simulink model "dft_polyphase_channelizer_4_by_2"  (R2018b)
settings: Solver=FixedStepDiscrete  StartTime=0.0  StopTime=t(end)  RelTol=1e-3  EnableMultiTasking=on
InitFcn:
  | M = 4; % Number of channels in the filter bank.
  | N = 8;  % Number of taps in each FIR filter.
  | n_out = 4000; % Number of output samples
  | datatypeselector = 'dsp'; % 'double' 'single' 'hdl' 'dsp'
  | fidatatype = 'Fixed'; % 'Fixed' 'ScaledDouble'
  | [T,B,U,b,u,t,fs] = generate_inputs(M,N,n_out,datatypeselector,fidatatype);
undefined symbols (not defined in the file or in its folder): B, fs, T
settings Model: Creator=tbryan  LastModifiedBy=tbryan
settings SolverCC: AutoInsertRateTranBlk=on
settings OptimizationCC: LifeSpan=inf
settings DebuggingCC: AllowSymbolicDim=off  LibraryContextMissingDiagnostic=none  SFUnexpectedBacktrackingDiag=warning  SFNoUnconditionalDefaultTransitionDiag=warning  SFExecutionAtInitializationDiag=none
settings SFSimCC: SimUseLocalCustomCode=off
settings RTWCC: RTWUseLocalCustomCode=off
settings CodeAppCC: StateflowObjectComments=on
settings GRTTargetCC: TargetLangStandard=C89/C90 (ANSI)  GeneratePreprocessorConditionals=Disable all
settings ConfigComp: CovMetricSettings=dw  CovHtmlReporting=on  CovSaveCumulativeToWorkspaceVar=on  CovSaveSingleToWorkspaceVar=on  CovExternalEMLEnable=off

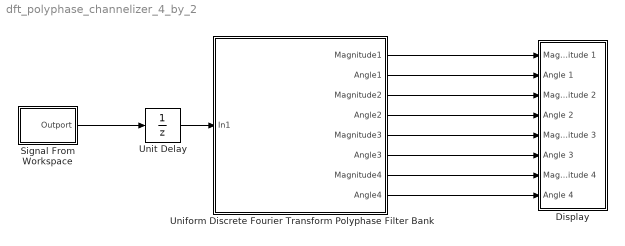
== system dft_polyphase_channelizer_4_by_2 ==
  Display : Subsystem
  Signal From Workspace : Subsystem  mask(Signal From Workspace){X=u, Ts=1/fs, nsamps=1, OutputAfterFinalValue=Setting to zero, ignoreOrWarnInputAndFrameLengths=off, OutputFrames=off}
      mask prompts: X "Signal:"; Ts "Sample time:"; nsamps "Samples per frame:"; OutputAfterFinalValue "Form output after final data value by:"; ignoreOrWarnInputAndFrameLengths "Warn when frame size does not evenly divide input length"; OutputFrames "Output Frames"
      mask help:
      | Output signal samples obtained from the MATLAB workspace at successive sample times.  A signal matrix is interpreted as having one channel per column.  Signal columns may be buffered into frames by specifying a number of samples per frame greater than 1.
      |
      | An M x N x P signal array outputs M x N matrices at successive sample times.  The samples per frame must be equal to 1 for three-dimensional signal arrays.
      mask init:
      | dispX = get_param(gcbh, 'X');
      | [s,Ts] = dspblksfw2('init', X,Ts,nsamps);
      mask Help: eval('blocksethelp');
      mask TypeOptions OutputAfterFinalValue: Setting to zero | Holding final value | Cyclic repetition
      mask Callback OutputAfterFinalValue: dspblksfw2
      mask Display: disp(dispX)
  Uniform Discrete Fourier Transform Polyphase Filter Bank : Subsystem
  Unit Delay : UnitDelay  SampleTime=-1
  wires:
  Signal From Workspace/1(Outport) -> Unit Delay/1
  Unit Delay/1 -> Uniform Discrete Fourier Transform Polyphase Filter Bank/1(In1)
  Uniform Discrete Fourier Transform Polyphase Filter Bank/1(Magnitude1) -> Display/1(Magnitude 1)
  Uniform Discrete Fourier Transform Polyphase Filter Bank/2(Angle1) -> Display/2(Angle 1)
  Uniform Discrete Fourier Transform Polyphase Filter Bank/3(Magnitude2) -> Display/3(Magnitude 2)
  Uniform Discrete Fourier Transform Polyphase Filter Bank/4(Angle2) -> Display/4(Angle 2)
  Uniform Discrete Fourier Transform Polyphase Filter Bank/5(Magnitude3) -> Display/5(Magnitude 3)
  Uniform Discrete Fourier Transform Polyphase Filter Bank/6(Angle3) -> Display/6(Angle 3)
  Uniform Discrete Fourier Transform Polyphase Filter Bank/7(Magnitude4) -> Display/7(Magnitude 4)
  Uniform Discrete Fourier Transform Polyphase Filter Bank/8(Angle4) -> Display/8(Angle 4)

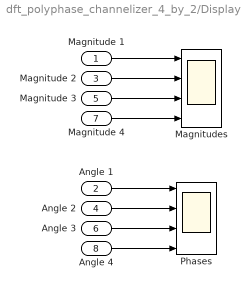
== system dft_polyphase_channelizer_4_by_2/Display ==
  Magnitude 1 : Inport
  Angle 1 : Inport  Port=2
  Magnitude 2 : Inport  Port=3
  Angle 2 : Inport  Port=4
  Magnitude 3 : Inport  Port=5
  Angle 3 : Inport  Port=6
  Magnitude 4 : Inport  Port=7
  Angle 4 : Inport  Port=8
  Magnitudes : Scope  NumInputPorts=4
  Phases : Scope  NumInputPorts=4
  wires:
  Angle 3/1 -> Phases/3
  Magnitude 2/1 -> Magnitudes/2
  Magnitude 1/1 -> Magnitudes/1
  Magnitude 4/1 -> Magnitudes/4
  Angle 2/1 -> Phases/2
  Angle 4/1 -> Phases/4
  Magnitude 3/1 -> Magnitudes/3
  Angle 1/1 -> Phases/1

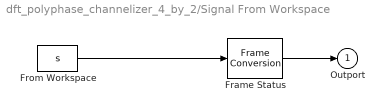
== system dft_polyphase_channelizer_4_by_2/Signal From Workspace ==
  Frame Status : FrameConversion  OutFrame=Sample-based
  From Workspace : FromWorkspace  VariableName=s  SampleTime=Ts  Interpolate=off  OutputAfterFinalValue=Setting to zero
  Outport : Outport  InitialOutput=0
  wires:
  Frame Status/1 -> Outport/1
  From Workspace/1 -> Frame Status/1

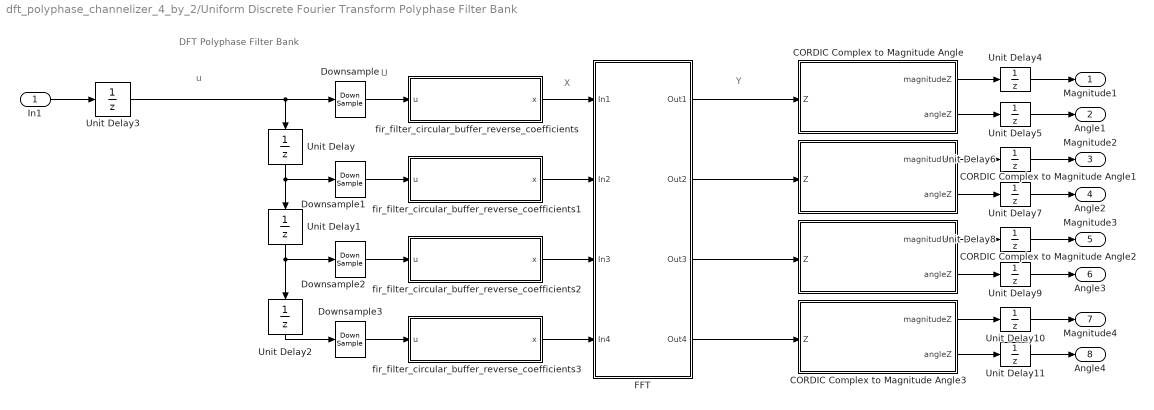
== system dft_polyphase_channelizer_4_by_2/Uniform Discrete Fourier Transform Polyphase Filter Bank ==
  note: DFT Polyphase Filter Bank
  note: U
  note: u
  note: X
  note: Y
  In1 : Inport
  " CORDIC Complex to Magnitude Angle" : MATLAB Function  TreatAsAtomicUnit=on
  " CORDIC Complex to Magnitude Angle1" : MATLAB Function  TreatAsAtomicUnit=on
  " CORDIC Complex to Magnitude Angle2" : MATLAB Function  TreatAsAtomicUnit=on
  " CORDIC Complex to Magnitude Angle3" : MATLAB Function  TreatAsAtomicUnit=on
  Downsample{,1..3} (4 alike) : DownSample  N=4  RateOptions=Allow multirate processing
  FFT : Subsystem
      mask Display: disp('IDFT')
  Unit Delay{,1..11} (12 alike) : UnitDelay  SampleTime=-1
  fir_filter_circular_buffer_reverse_coefficients : MATLAB Function  TreatAsAtomicUnit=on  mask{b=B(1,:), T=T.fir_filter}
      mask prompts: b "Coefficients: b from MATLAB's filter(b,1,x)"
  fir_filter_circular_buffer_reverse_coefficients1 : MATLAB Function  TreatAsAtomicUnit=on  mask{b=B(2,:), T=T.fir_filter}
      mask prompts: b "Coefficients: b from MATLAB's filter(b,1,x)"
  fir_filter_circular_buffer_reverse_coefficients2 : MATLAB Function  TreatAsAtomicUnit=on  mask{b=B(3,:), T=T.fir_filter}
      mask prompts: b "Coefficients: b from MATLAB's filter(b,1,x)"
  fir_filter_circular_buffer_reverse_coefficients3 : MATLAB Function  TreatAsAtomicUnit=on  mask{b=B(4,:), T=T.fir_filter}
      mask prompts: b "Coefficients: b from MATLAB's filter(b,1,x)"
  Magnitude1 : Outport
  Angle1 : Outport  Port=2
  Magnitude2 : Outport  Port=3
  Angle2 : Outport  Port=4
  Magnitude3 : Outport  Port=5
  Angle3 : Outport  Port=6
  Magnitude4 : Outport  Port=7
  Angle4 : Outport  Port=8
  wires:
  FFT/1(Out1) -> " CORDIC Complex to Magnitude Angle"/1(Z)
  FFT/2(Out2) -> " CORDIC Complex to Magnitude Angle1"/1(Z)
  FFT/3(Out3) -> " CORDIC Complex to Magnitude Angle2"/1(Z)
  FFT/4(Out4) -> " CORDIC Complex to Magnitude Angle3"/1(Z)
  Unit Delay1/1 -> Unit Delay2/1, Downsample2/1
  fir_filter_circular_buffer_reverse_coefficients1/1(x) -> FFT/2(In2)
  Unit Delay/1 -> Unit Delay1/1, Downsample1/1
  fir_filter_circular_buffer_reverse_coefficients/1(x) -> FFT/1(In1)
  fir_filter_circular_buffer_reverse_coefficients2/1(x) -> FFT/3(In3)
  Unit Delay2/1 -> Downsample3/1
  fir_filter_circular_buffer_reverse_coefficients3/1(x) -> FFT/4(In4)
  Downsample3/1 -> fir_filter_circular_buffer_reverse_coefficients3/1(u)
  Downsample2/1 -> fir_filter_circular_buffer_reverse_coefficients2/1(u)
  Downsample1/1 -> fir_filter_circular_buffer_reverse_coefficients1/1(u)
  Downsample/1 -> fir_filter_circular_buffer_reverse_coefficients/1(u)
  In1/1 -> Unit Delay3/1
  Unit Delay3/1 -> Unit Delay/1, Downsample/1
  Unit Delay4/1 -> Magnitude1/1
  " CORDIC Complex to Magnitude Angle"/1(magnitudeZ) -> Unit Delay4/1
  Unit Delay5/1 -> Angle1/1
  " CORDIC Complex to Magnitude Angle"/2(angleZ) -> Unit Delay5/1
  Unit Delay6/1 -> Magnitude2/1
  " CORDIC Complex to Magnitude Angle1"/1(magnitudeZ) -> Unit Delay6/1
  Unit Delay7/1 -> Angle2/1
  " CORDIC Complex to Magnitude Angle1"/2(angleZ) -> Unit Delay7/1
  Unit Delay8/1 -> Magnitude3/1
  " CORDIC Complex to Magnitude Angle2"/1(magnitudeZ) -> Unit Delay8/1
  Unit Delay9/1 -> Angle3/1
  " CORDIC Complex to Magnitude Angle2"/2(angleZ) -> Unit Delay9/1
  Unit Delay10/1 -> Magnitude4/1
  " CORDIC Complex to Magnitude Angle3"/1(magnitudeZ) -> Unit Delay10/1
  Unit Delay11/1 -> Angle4/1
  " CORDIC Complex to Magnitude Angle3"/2(angleZ) -> Unit Delay11/1

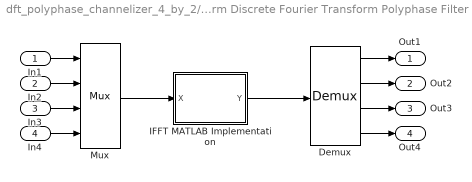
== system dft_polyphase_channelizer_4_by_2/Uniform Discrete Fourier Transform Polyphase Filter Bank/FFT ==
  In1 : Inport
  In2 : Inport  Port=2
  In3 : Inport  Port=3
  In4 : Inport  Port=4
  Demux : Demux
  IFFT MATLAB Implementation : MATLAB Function  TreatAsAtomicUnit=on  mask{T=T.fft}
      mask prompts: T "Types table"
  Mux : Mux
  Out1 : Outport
  Out2 : Outport  Port=2
  Out3 : Outport  Port=3
  Out4 : Outport  Port=4
  wires:
  Mux/1 -> IFFT MATLAB Implementation/1(X)
  IFFT MATLAB Implementation/1(Y) -> Demux/1
  In1/1 -> Mux/1
  In4/1 -> Mux/4
  In3/1 -> Mux/3
  In2/1 -> Mux/2
  Demux/2 -> Out2/1
  Demux/3 -> Out3/1
  Demux/4 -> Out4/1
  Demux/1 -> Out1/1

== matlab function dft_polyphase_channelizer_4_by_2/Uniform Discrete Fourier Transform Polyphase Filter Bank/ CORDIC Complex to Magnitude Angle1 ==
  data: Z input; magnitudeZ output; angleZ output
function [magnitudeZ, angleZ] = cordic_magnitude_angle(Z)
    [magnitudeZ, angleZ] = cordic_cart2pol(Z);
end

== matlab function dft_polyphase_channelizer_4_by_2/Uniform Discrete Fourier Transform Polyphase Filter Bank/ CORDIC Complex to Magnitude Angle ==
  data: Z input; magnitudeZ output; angleZ output
function [magnitudeZ, angleZ] = cordic_magnitude_angle(Z)
    [magnitudeZ, angleZ] = cordic_cart2pol(Z);
end

== matlab function dft_polyphase_channelizer_4_by_2/Uniform Discrete Fourier Transform Polyphase Filter Bank/ CORDIC Complex to Magnitude Angle2 ==
  data: Z input; magnitudeZ output; angleZ output
function [magnitudeZ, angleZ] = cordic_magnitude_angle(Z)
    [magnitudeZ, angleZ] = cordic_cart2pol(Z);
end

== matlab function dft_polyphase_channelizer_4_by_2/Uniform Discrete Fourier Transform Polyphase Filter Bank/ CORDIC Complex to Magnitude Angle3 ==
  data: Z input; magnitudeZ output; angleZ output
function [magnitudeZ, angleZ] = cordic_magnitude_angle(Z)
    [magnitudeZ, angleZ] = cordic_cart2pol(Z);
end

== matlab function dft_polyphase_channelizer_4_by_2/Uniform Discrete Fourier Transform Polyphase Filter Bank/FFT/IFFT MATLAB Implementation ==
  data: X input; Y output; T parameter
function Y = inverse_fft_block(X,T)
    dim = 1;
    Y = inverse_fft(X, T, dim);
end

== matlab function dft_polyphase_channelizer_4_by_2/Uniform Discrete Fourier Transform Polyphase Filter Bank/fir_filter_circular_buffer_reverse_coefficients ==
  data: u input; x output; b parameter; T parameter
function x = fir_filter(u, b, T)
    persistent p z
    if isempty(p)
        p = zeros(1,'like',T.p);
        z = zeros(size(b),'like',T.z);
    end
    [x,z,p] = fir_filter_circular_buffer(b,u,z,p,T);
end

== matlab function dft_polyphase_channelizer_4_by_2/Uniform Discrete Fourier Transform Polyphase Filter Bank/fir_filter_circular_buffer_reverse_coefficients1 ==
  data: u input; x output; b parameter; T parameter
function x = fir_filter(u, b, T)
    persistent p z
    if isempty(p)
        p = zeros(1,'like',T.p);
        z = zeros(size(b),'like',T.z);
    end
    [x,z,p] = fir_filter_circular_buffer(b,u,z,p,T);
end

== matlab function dft_polyphase_channelizer_4_by_2/Uniform Discrete Fourier Transform Polyphase Filter Bank/fir_filter_circular_buffer_reverse_coefficients2 ==
  data: u input; x output; b parameter; T parameter
function x = fir_filter(u, b, T)
    persistent p z
    if isempty(p)
        p = zeros(1,'like',T.p);
        z = zeros(size(b),'like',T.z);
    end
    [x,z,p] = fir_filter_circular_buffer(b,u,z,p,T);
end

== matlab function dft_polyphase_channelizer_4_by_2/Uniform Discrete Fourier Transform Polyphase Filter Bank/fir_filter_circular_buffer_reverse_coefficients3 ==
  data: u input; x output; b parameter; T parameter
function x = fir_filter(u, b, T)
    persistent p z
    if isempty(p)
        p = zeros(1,'like',T.p);
        z = zeros(size(b),'like',T.z);
    end
    [x,z,p] = fir_filter_circular_buffer(b,u,z,p,T);
end
